simulink model "pmsm_smo"  (R2024b)
settings: Solver=FixedStepDiscrete  StartTime=0.0  StopTime=15  FixedStep=50e-6  RelTol=1e-3  EnableMultiTasking=on
values from neighbouring files (symbols this model uses):
  CalibId = 0    [mchp_pmsm_foc_smo_dsPIC33_data.m]
  CalibIq = 1    [mchp_pmsm_foc_smo_dsPIC33_data.m]
  CalibSpeed = 500    [mchp_pmsm_foc_smo_dsPIC33_data.m]
  CalibTime = 1/CalibFreq    (= 0.12)    [mchp_pmsm_foc_smo_dsPIC33_data.m]
  CalibVd = -0.7    [mchp_pmsm_foc_smo_dsPIC33_data.m]
  CalibVq = 2.69    [mchp_pmsm_foc_smo_dsPIC33_data.m]
  PI_Ki_id = (6.60e2)*Ts    (= 0.033)    [mchp_pmsm_foc_smo_dsPIC33_data.m]
  PI_Ki_iq = (6.60e2)*Ts    (= 0.033)    [mchp_pmsm_foc_smo_dsPIC33_data.m]
  PI_Ki_speed = (1.96e-6)    (= 1.96e-06)    [mchp_pmsm_foc_smo_dsPIC33_data.m]
  PI_Kp_id = 0.852    [mchp_pmsm_foc_smo_dsPIC33_data.m]
  PI_Kp_iq = 0.852    [mchp_pmsm_foc_smo_dsPIC33_data.m]
  PI_Kp_speed = 0.0062756    [mchp_pmsm_foc_smo_dsPIC33_data.m]
  PWM_frequency = 20e3    (= 20000)    [mchp_pmsm_foc_smo_dsPIC33_data.m]
  Ts = T_pwm    (= 5e-05)    [mchp_pmsm_foc_smo_dsPIC33_data.m]
  Ts_serialIn = 100e-3    (= 0.1)    [mchp_pmsm_foc_smo_dsPIC33_data.m]
  Ts_speed = 30*Ts    (= 0.0015)    [mchp_pmsm_foc_smo_dsPIC33_data.m]
undefined symbols (not defined in the file or in its folder): A0, A4, ADC, B0, C10, C11, C6, C7, C8, D11, D12, DiscIntNeverNeededParam, inverter, Max, MaxPer, ms, NumBits1, NumBits2, OpMode, P1, P17, P20, P39, P40, P41, P43, P44, P60, P61, Pin, pmsm, PWM1_Trg1, Resol, s, target, us
libraries: simulink x39, MCHP_Blockset x22, mcbcontrolslib x14, slpidlib x5
(part 4 of 5)

== system pmsm_smo/BOARD MCLV-48V-300W dsPIC33AK128MC106 MC DIM/Downsample Averaged x20 ==
  note: DownSample & Average by changing data scaling
  In1 : Inport
  Compare To Constant : simulink/Logic and Bit Operations/Compare To Constant  relop===  const=1  OutDataTypeStr=boolean
  Counter Limited : simulink/Sources/Counter Limited  uplimit=DownSample-1  tsamp=-1
  Data Type Duplicate : DataTypeDuplicate
  Data Type Propagation : simulink/Signal Attributes/Data Type Propagation  PropDataType=fixdt(1, 16)  IfRefDouble=double  IfRefSingle=single  IsSigned=IsSigned1 or IsSigned2  NumBitsBase=NumBits1+NumBits2  NumBitsMult=1  NumBitsAdd=0  NumBitsAllowFinal=-1  PropScaling=2^-10  ValuesUsedBestPrec=[5 -7]  SlopeBase=Slope1  SlopeMult=1  SlopeAdd=0  BiasBase=Bias1  BiasMult=1  BiasAdd=0
  Data Type Propagation1 : simulink/Signal Attributes/Data Type Propagation  PropDataType=fixdt(1, 16)  IfRefDouble=double  IfRefSingle=single  IsSigned=IsSigned1 or IsSigned2  NumBitsBase=NumBits1+NumBits2  NumBitsMult=1  NumBitsAdd=0  NumBitsAllowFinal=-1  PropScaling=2^-10  ValuesUsedBestPrec=[5 -7]  SlopeBase=PosRange1  SlopeMult=1  SlopeAdd=0  BiasBase=Bias1  BiasMult=1  BiasAdd=0
  Discrete-Time Integrator : DiscreteIntegrator  IntegratorMethod=Accumulation: Backward Euler  gainval=1  ExternalReset=sampled level  SampleTime=-1  OutDataTypeStr=Inherit: Inherit via back propagation  ICPrevOutput=DiscIntNeverNeededParam  ICPrevScaledInput=DiscIntNeverNeededParam
  Gain : Gain  Gain=1/DownSample  OutDataTypeStr=Inherit: Inherit via back propagation  RndMeth=Round
  Gain1 : Gain  Gain=1/DownSample  OutDataTypeStr=Inherit: Inherit via back propagation
  Rate Transition1 : RateTransition  OutPortSampleTimeOpt=Multiple of input port sample time  OutPortSampleTimeMultiple=DownSample  OutPortSampleTime=DownSample
  Rate Transition3 : RateTransition  OutPortSampleTimeOpt=Multiple of input port sample time  OutPortSampleTimeMultiple=DownSample  OutPortSampleTime=DownSample
  Terminator : Terminator
  Out1 : Outport  VectorParamsAs1DForOutWhenUnconnected=off
  wires:
  Gain1/1 -> Data Type Propagation1/3, Terminator/1
  Rate Transition1/1 -> Data Type Duplicate/1, Data Type Propagation1/1, Data Type Propagation1/2
  Gain/1 -> Out1/1, Data Type Duplicate/2
  Counter Limited/1 -> Compare To Constant/1
  Discrete-Time Integrator/1 -> Rate Transition3/1, Data Type Propagation/3
  Compare To Constant/1 -> Discrete-Time Integrator/2
  In1/1 -> Data Type Propagation/1, Data Type Propagation/2, Discrete-Time Integrator/1, Rate Transition1/1
  Rate Transition3/1 -> Gain/1, Gain1/1

== system pmsm_smo/BOARD MCLV-48V-300W dsPIC33AK128MC106 MC DIM/Downsample x20 ==
  note: DownSample & Average by changing data scaling
  In1 : Inport
  Compare To Constant : simulink/Logic and Bit Operations/Compare To Constant  relop===  const=1  OutDataTypeStr=boolean
  Counter Limited : simulink/Sources/Counter Limited  uplimit=DownSample-1  tsamp=-1
  Data Type Duplicate : DataTypeDuplicate
  Data Type Propagation : simulink/Signal Attributes/Data Type Propagation  PropDataType=fixdt(1, 16)  IfRefDouble=double  IfRefSingle=single  IsSigned=IsSigned1 or IsSigned2  NumBitsBase=NumBits1+NumBits2  NumBitsMult=1  NumBitsAdd=0  NumBitsAllowFinal=-1  PropScaling=2^-10  ValuesUsedBestPrec=[5 -7]  SlopeBase=Slope1  SlopeMult=1  SlopeAdd=0  BiasBase=Bias1  BiasMult=1  BiasAdd=0
  Data Type Propagation1 : simulink/Signal Attributes/Data Type Propagation  PropDataType=fixdt(1, 16)  IfRefDouble=double  IfRefSingle=single  IsSigned=IsSigned1 or IsSigned2  NumBitsBase=NumBits1+NumBits2  NumBitsMult=1  NumBitsAdd=0  NumBitsAllowFinal=-1  PropScaling=2^-10  ValuesUsedBestPrec=[5 -7]  SlopeBase=PosRange1  SlopeMult=1  SlopeAdd=0  BiasBase=Bias1  BiasMult=1  BiasAdd=0
  Discrete-Time Integrator : DiscreteIntegrator  IntegratorMethod=Accumulation: Backward Euler  gainval=1  ExternalReset=sampled level  SampleTime=-1  OutDataTypeStr=Inherit: Inherit via back propagation  ICPrevOutput=DiscIntNeverNeededParam  ICPrevScaledInput=DiscIntNeverNeededParam
  Gain : Gain  Gain=1/DownSample  OutDataTypeStr=Inherit: Inherit via back propagation  RndMeth=Round
  Gain1 : Gain  Gain=1/DownSample  OutDataTypeStr=Inherit: Inherit via back propagation
  Rate Transition1 : RateTransition  OutPortSampleTimeOpt=Multiple of input port sample time  OutPortSampleTimeMultiple=DownSample  OutPortSampleTime=DownSample
  Rate Transition3 : RateTransition  OutPortSampleTimeOpt=Multiple of input port sample time  OutPortSampleTimeMultiple=DownSample  OutPortSampleTime=DownSample
  Terminator : Terminator
  Out1 : Outport  VectorParamsAs1DForOutWhenUnconnected=off
  wires:
  Rate Transition3/1 -> Gain1/1, Gain/1
  In1/1 -> Rate Transition1/1, Discrete-Time Integrator/1, Data Type Propagation/2, Data Type Propagation/1
  Compare To Constant/1 -> Discrete-Time Integrator/2
  Discrete-Time Integrator/1 -> Data Type Propagation/3, Rate Transition3/1
  Counter Limited/1 -> Compare To Constant/1
  Gain/1 -> Data Type Duplicate/2, Out1/1
  Rate Transition1/1 -> Data Type Propagation1/2, Data Type Propagation1/1, Data Type Duplicate/1
  Gain1/1 -> Terminator/1, Data Type Propagation1/3

== system pmsm_smo/BOARD MCLV-48V-300W dsPIC33AK128MC106 MC DIM/Downsample x20 _ ==
  note: DownSample & Average by changing data scaling
  In1 : Inport
  Compare To Constant : simulink/Logic and Bit Operations/Compare To Constant  relop===  const=1  OutDataTypeStr=boolean
  Counter Limited : simulink/Sources/Counter Limited  uplimit=DownSample-1  tsamp=-1
  Data Type Duplicate : DataTypeDuplicate
  Data Type Propagation : simulink/Signal Attributes/Data Type Propagation  PropDataType=fixdt(1, 16)  IfRefDouble=double  IfRefSingle=single  IsSigned=IsSigned1 or IsSigned2  NumBitsBase=NumBits1+NumBits2  NumBitsMult=1  NumBitsAdd=0  NumBitsAllowFinal=-1  PropScaling=2^-10  ValuesUsedBestPrec=[5 -7]  SlopeBase=Slope1  SlopeMult=1  SlopeAdd=0  BiasBase=Bias1  BiasMult=1  BiasAdd=0
  Data Type Propagation1 : simulink/Signal Attributes/Data Type Propagation  PropDataType=fixdt(1, 16)  IfRefDouble=double  IfRefSingle=single  IsSigned=IsSigned1 or IsSigned2  NumBitsBase=NumBits1+NumBits2  NumBitsMult=1  NumBitsAdd=0  NumBitsAllowFinal=-1  PropScaling=2^-10  ValuesUsedBestPrec=[5 -7]  SlopeBase=PosRange1  SlopeMult=1  SlopeAdd=0  BiasBase=Bias1  BiasMult=1  BiasAdd=0
  Discrete-Time Integrator : DiscreteIntegrator  IntegratorMethod=Accumulation: Backward Euler  gainval=1  ExternalReset=sampled level  SampleTime=-1  OutDataTypeStr=Inherit: Inherit via back propagation  ICPrevOutput=DiscIntNeverNeededParam  ICPrevScaledInput=DiscIntNeverNeededParam
  Gain : Gain  Gain=1/DownSample  OutDataTypeStr=Inherit: Inherit via back propagation  RndMeth=Round
  Gain1 : Gain  Gain=1/DownSample  OutDataTypeStr=Inherit: Inherit via back propagation
  Rate Transition1 : RateTransition  OutPortSampleTimeOpt=Multiple of input port sample time  OutPortSampleTimeMultiple=DownSample  OutPortSampleTime=DownSample
  Rate Transition3 : RateTransition  OutPortSampleTimeOpt=Multiple of input port sample time  OutPortSampleTimeMultiple=DownSample  OutPortSampleTime=DownSample
  Terminator : Terminator
  Out1 : Outport  VectorParamsAs1DForOutWhenUnconnected=off
  wires:
  Gain1/1 -> Data Type Propagation1/3, Terminator/1
  Rate Transition1/1 -> Data Type Duplicate/1, Data Type Propagation1/1, Data Type Propagation1/2
  Gain/1 -> Out1/1, Data Type Duplicate/2
  Counter Limited/1 -> Compare To Constant/1
  Discrete-Time Integrator/1 -> Rate Transition3/1, Data Type Propagation/3
  Compare To Constant/1 -> Discrete-Time Integrator/2
  In1/1 -> Data Type Propagation/1, Data Type Propagation/2, Discrete-Time Integrator/1, Rate Transition1/1
  Rate Transition3/1 -> Gain/1, Gain1/1

== system pmsm_smo/BOARD MCLV-48V-300W dsPIC33AK128MC106 MC DIM/MCLV 48V-300W board webpage ==

== system pmsm_smo/BOARD MCLV-48V-300W dsPIC33AK128MC106 MC DIM/Timing Analysis ==
  note: CPU overload is 0 if no overload took place between two MCU Overload block execution.
      | Otherwise, bits field output code for TID(s) responsible for at least one overload.
  Downsample Averaged2 : Subsystem  mask{InputSampleTime=.0005, DownSample=200}
      mask prompts: InputSampleTime "Input sample time"; DownSample "DownSample Factor"
  Gain : Gain  Gain=5e-9/.0005 * 100  OutMin=0  OutMax=100  OutDataTypeStr=fixdt(0,16)  RndMeth=Simplest  SaturateOnIntegerOverflow=on
  MCU Load : MCHP_Blockset/Profiling/MCU Load  MCULoadPin_TXT=None  MCULoadMeasure=on  TIMER_Resolution_TXT="Resol: 0.005(us)  -  Max: 0.328(ms)"  MCHP_TIMER_REQUEST={MCU_Load}{MCU_Load}21:5:0:0:[]:32768;  MCHP_TIMER_RESULT=[2 65535 ]  MCHP_MASTERLINK=pmsm_smo/BOARD MCLV-48V-300W dsPIC33AK128MC106 MC DIM/Microchip Master  MCHP_COMPILED_INFO="CompiledSampleTime= [0.00050000000000000001041   0 ];CompiledInportDataTypes=[    ];CompiledInportDataWidth=[];"  Info="Timer 2:  Resol: 5(ns)  -  Max: 327.68(us)"  SampleTime=.0005
      settings: SourceProductName=MPLAB Device Blocks for Simulink
  MCU Overload : MCHP_Blockset/Profiling/MCU Overload  MCUOverloadBlockOutput=on  MCUOverLoadPin_TXT=None  MCHP_MASTERLINK=pmsm_smo/BOARD MCLV-48V-300W dsPIC33AK128MC106 MC DIM/Microchip Master  SampleTime=-1
      settings: SourceProductName=MPLAB Device Blocks for Simulink
  Overload : Constant  Value=65535  OutDataTypeStr=Inherit: Inherit via back propagation
  Rate Transition : RateTransition  Deterministic=off  OutPortSampleTime=.0005*200
  Switch : Switch  Criteria=u2 ~= 0  SaturateOnIntegerOverflow=off  InputSameDT=off
  CPU Load : Outport  Unit=%  SampleTime=.0005*200
  CPU Overload : Outport  Port=2
  wires:
  Rate Transition/1 -> Switch/2
  MCU Overload/1 -> Rate Transition/1, CPU Overload/1
  MCU Load/1 -> Downsample Averaged2/1(In1)
  Downsample Averaged2/1(Out1) -> Switch/3
  Switch/1 -> Gain/1
  Overload/1 -> Switch/1
  Gain/1 -> CPU Load/1

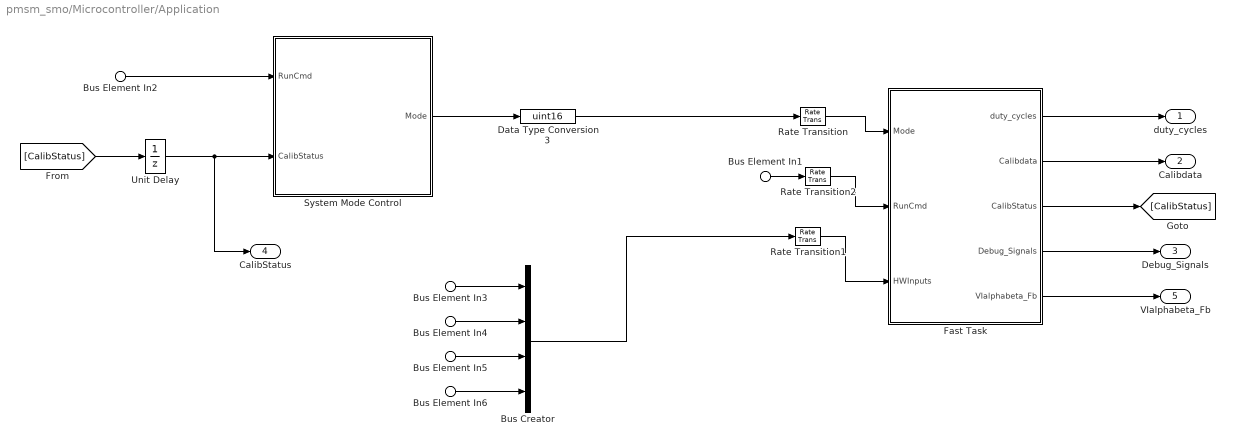
== system pmsm_smo/Microcontroller/Application ==
  Bus Element In3 : Inport  PortName=Currents  Element=Iab
  Bus Element In4 : Inport  Port=2  PortName=PositionAndSpeed  Element=Theta_SMO
  Bus Element In6 : Inport  Port=2  PortName=PositionAndSpeed  Element=Speed_SMO
  Bus Element In1 : Inport  Port=3  PortName=Commands  Element=RunCmd
  Bus Element In2 : Inport  Port=3  PortName=Commands  Element=RunCmd
  Bus Element In5 : Inport  Port=3  PortName=Commands  Element=SpeedRef
  Bus Creator : BusCreator  Inputs=4
  Data Type Conversion3 : DataTypeConversion  OutDataTypeStr=uint16  RndMeth=Simplest  SaturateOnIntegerOverflow=off
  Fast Task : Subsystem
  Rate Transition : RateTransition  Deterministic=off  OutPortSampleTime=Ts
  Rate Transition1 : RateTransition  Deterministic=off  OutPortSampleTime=Ts
  Rate Transition2 : RateTransition  Deterministic=off  OutPortSampleTime=Ts
  System Mode Control : Subsystem
  Unit Delay : UnitDelay  SampleTime=-1  HasFrameUpgradeWarning=on
  duty_cycles : Outport  VectorParamsAs1DForOutWhenUnconnected=off
  Calibdata : Outport  Port=2
  Debug_Signals : Outport  Port=3
  CalibStatus : Outport  Port=4
  VIalphabeta_Fb : Outport  Port=5
  wires:
  System Mode Control/1(Mode) -> Data Type Conversion3/1
  Data Type Conversion3/1 -> Rate Transition/1
  Rate Transition/1 -> Fast Task/1(Mode)
  Bus Element In1/1 -> Rate Transition2/1
  Fast Task/1(duty_cycles) -> duty_cycles/1
  Bus Element In2/1 -> System Mode Control/1(RunCmd)
  Fast Task/3(CalibStatus) -> [CalibStatus]
  [CalibStatus] -> Unit Delay/1
  Bus Element In3/1 -> Bus Creator/1
  Bus Element In4/1 -> Bus Creator/2
  Bus Element In5/1 -> Bus Creator/3
  Bus Element In6/1 -> Bus Creator/4
  Bus Creator/1 -> Rate Transition1/1
  Rate Transition1/1 -> Fast Task/3(HWInputs)
  Rate Transition2/1 -> Fast Task/2(RunCmd)
  Unit Delay/1 -> CalibStatus/1, System Mode Control/2(CalibStatus)
  Fast Task/2(Calibdata) -> Calibdata/1
  Fast Task/4(Debug_Signals) -> Debug_Signals/1
  Fast Task/5(VIalphabeta_Fb) -> VIalphabeta_Fb/1

== system pmsm_smo/Microcontroller/Application_Abstraction ==
  Iab_Measured : Inport
  calibdata : Inport  Port=2
  VIalphabeta_Fb : Inport  Port=3
  Commands : Inport  Port=4
  Bus Creator : BusCreator  Inputs=1
  Bus Creator1 : BusCreator  Inputs=2
  SMO : Subsystem
  Currents : Outport
  PositionAndSpeed : Outport  Port=2
  wires:
  Bus Creator1/1 -> PositionAndSpeed/1
  Iab_Measured/1 -> Bus Creator/1  "Iab"
  Bus Creator/1 -> Currents/1
  Commands/1 -> SMO/2(Commands)
  VIalphabeta_Fb/1 -> SMO/1(VIalphabeta_Fb)
  SMO/1(Speed_meas) -> Bus Creator1/1  "Speed_SMO"
  SMO/2(Pos_PU) -> Bus Creator1/2  "Theta_SMO"
  calibdata/1 -> SMO/3(calibdata)

== system pmsm_smo/Microcontroller/Command_Signals ==
  note: Subsystem
  Command_Data : Inport
  Bus Creator : BusCreator  Inputs=2
  Command Signals : Subsystem  Variant=on  VariantControlMode=sim codegen switching
  Commands : Outport
  wires:
  Bus Creator/1 -> Commands/1
  Command Signals/1(RunCmd) -> Bus Creator/1  "RunCmd"
  Command Signals/2(SpeedRef) -> Bus Creator/2  "SpeedRef"
  Command_Data/1 -> Command Signals/1(Command_Data)

== system pmsm_smo/Microcontroller/Data Monitoring ==
  Data_Monitor : Inport
  Constant : Constant  OutDataTypeStr=boolean
  Rate Transition13 : RateTransition  Deterministic=off  OutPortSampleTime=Ts_serialIn
  Rate Transition14 : RateTransition  Deterministic=off  OutPortSampleTime=Ts_serialOut
  Rate Transition15 : RateTransition  Deterministic=off  OutPortSampleTime=Ts_serialOut
  SerialInDrivers : Subsystem
  SerialOutDrivers : Subsystem  Variant=on  VariantControlMode=sim codegen switching
  Subsystem Reference : Subsystem  TreatAsAtomicUnit=on  ReferencedSubsystem=SCIOutAbstractionFocQep
  Subsystem Reference1 : Subsystem  TreatAsAtomicUnit=on  ReferencedSubsystem=SCIInAbstractionFocQep
  Terminator : Terminator
  wires:
  Subsystem Reference1/1 -> Terminator/1
  Constant/1 -> Rate Transition13/1
  Rate Transition15/1 -> Subsystem Reference/1
  Rate Transition14/1 -> Subsystem Reference/2
  Subsystem Reference1/2 -> Rate Transition15/1
  Rate Transition13/1 -> Subsystem Reference1/2
  Subsystem Reference/1 -> SerialOutDrivers/1(SerialData)
  SerialInDrivers/1(SCI_Data) -> Subsystem Reference1/1  "sci data 8 bytes"
  Data_Monitor/1 -> Rate Transition14/1

== system pmsm_smo/Microcontroller/Sensor_Signals ==
  note: 1) Add Subsystem or Model blocks as valid variant choices.
      | 2) You cannot connect blocks at this level. At simulation, connectivity is automatically
      | determined, based on the active variant and port name matching.
  Sim_In : Inport
  Codegen_in : Inport  Port=2
  Codegen : Subsystem  VariantControl=(codegen)
  sim : Subsystem  VariantControl=(sim)
  Sensor_signals : Outport

== system pmsm_smo/BOARD MCLV-48V-300W dsPIC33AK128MC106 MC DIM/Center & sign reversal/Downsample Averaged 2000 samples remove bias ==
  note: DownSample & Average by changing data scaling
  In1 : Inport
  Enable : EnablePort
  Compare To Constant : simulink/Logic and Bit Operations/Compare To Constant  relop===  const=1  OutDataTypeStr=boolean
  Counter Limited : simulink/Sources/Counter Limited  uplimit=DownSample-1  tsamp=-1
  Data Type Duplicate : DataTypeDuplicate
  Data Type Propagation : simulink/Signal Attributes/Data Type Propagation  PropDataType=fixdt(1, 16)  IfRefDouble=double  IfRefSingle=single  IsSigned=IsSigned1 or IsSigned2  NumBitsBase=NumBits1+NumBits2  NumBitsMult=1  NumBitsAdd=0  NumBitsAllowFinal=-1  PropScaling=2^-10  ValuesUsedBestPrec=[5 -7]  SlopeBase=Slope1  SlopeMult=1  SlopeAdd=0  BiasBase=Bias1  BiasMult=1  BiasAdd=0
  Data Type Propagation1 : simulink/Signal Attributes/Data Type Propagation  PropDataType=fixdt(1, 16)  IfRefDouble=double  IfRefSingle=single  IsSigned=IsSigned1 or IsSigned2  NumBitsBase=NumBits1+NumBits2  NumBitsMult=1  NumBitsAdd=0  NumBitsAllowFinal=-1  PropScaling=2^-10  ValuesUsedBestPrec=[5 -7]  SlopeBase=PosRange1  SlopeMult=1  SlopeAdd=0  BiasBase=Bias1  BiasMult=1  BiasAdd=0
  Discrete-Time Integrator : DiscreteIntegrator  IntegratorMethod=Accumulation: Backward Euler  gainval=1  ExternalReset=sampled level  SampleTime=-1  OutDataTypeStr=Inherit: Inherit via back propagation  ICPrevOutput=DiscIntNeverNeededParam  ICPrevScaledInput=DiscIntNeverNeededParam
  Gain : Gain  Gain=1/DownSample  OutDataTypeStr=uint16  RndMeth=Round
  Gain1 : Gain  Gain=1/DownSample  OutDataTypeStr=Inherit: Inherit via back propagation
  Gain2 : Gain  OutDataTypeStr=int32
  Rate Transition1 : RateTransition  OutPortSampleTimeOpt=Multiple of input port sample time  OutPortSampleTimeMultiple=DownSample  OutPortSampleTime=DownSample
  Rate Transition3 : RateTransition  OutPortSampleTimeOpt=Multiple of input port sample time  OutPortSampleTimeMultiple=DownSample  OutPortSampleTime=DownSample
  Terminator : Terminator
  Out1 : Outport  InitialOutput=[32768]  VectorParamsAs1DForOutWhenUnconnected=off
  wires:
  Gain1/1 -> Gain2/1, Data Type Propagation1/3  "Offset"
  Rate Transition1/1 -> Data Type Duplicate/1, Data Type Propagation1/1, Data Type Propagation1/2
  Gain/1 -> Terminator/1, Data Type Duplicate/2  "Offset_Value_Uint16"
  Counter Limited/1 -> Compare To Constant/1
  Discrete-Time Integrator/1 -> Rate Transition3/1, Data Type Propagation/3  "Intergrator_Out"
  Compare To Constant/1 -> Discrete-Time Integrator/2
  In1/1 -> Data Type Propagation/1, Data Type Propagation/2, Discrete-Time Integrator/1, Rate Transition1/1
  Rate Transition3/1 -> Gain/1, Gain1/1
  Gain2/1 -> Out1/1  "Offset_Value_int32"

== system pmsm_smo/BOARD MCLV-48V-300W dsPIC33AK128MC106 MC DIM/Timing Analysis/Downsample Averaged2 ==
  note: DownSample & Average by changing data scaling
  In1 : Inport
  Compare To Constant : simulink/Logic and Bit Operations/Compare To Constant  relop===  const=1  OutDataTypeStr=boolean
  Counter Limited : simulink/Sources/Counter Limited  uplimit=DownSample-1  tsamp=-1
  Data Type Duplicate : DataTypeDuplicate
  Data Type Propagation : simulink/Signal Attributes/Data Type Propagation  PropDataType=fixdt(1, 16)  IfRefDouble=double  IfRefSingle=single  IsSigned=IsSigned1 or IsSigned2  NumBitsBase=NumBits1+NumBits2  NumBitsMult=1  NumBitsAdd=0  NumBitsAllowFinal=-1  PropScaling=2^-10  ValuesUsedBestPrec=[5 -7]  SlopeBase=Slope1  SlopeMult=1  SlopeAdd=0  BiasBase=Bias1  BiasMult=1  BiasAdd=0
  Data Type Propagation1 : simulink/Signal Attributes/Data Type Propagation  PropDataType=fixdt(1, 16)  IfRefDouble=double  IfRefSingle=single  IsSigned=IsSigned1 or IsSigned2  NumBitsBase=NumBits1+NumBits2  NumBitsMult=1  NumBitsAdd=0  NumBitsAllowFinal=-1  PropScaling=2^-10  ValuesUsedBestPrec=[5 -7]  SlopeBase=PosRange1  SlopeMult=1  SlopeAdd=0  BiasBase=Bias1  BiasMult=1  BiasAdd=0
  Discrete-Time Integrator : DiscreteIntegrator  IntegratorMethod=Accumulation: Backward Euler  gainval=1  ExternalReset=sampled level  SampleTime=-1  OutDataTypeStr=Inherit: Inherit via back propagation  ICPrevOutput=DiscIntNeverNeededParam  ICPrevScaledInput=DiscIntNeverNeededParam
  Gain : Gain  Gain=1/DownSample  OutDataTypeStr=Inherit: Inherit via back propagation
  Gain1 : Gain  Gain=1/DownSample  OutDataTypeStr=Inherit: Inherit via back propagation
  Rate Transition1 : RateTransition  Deterministic=off  OutPortSampleTime=[InputSampleTime * DownSample]
  Rate Transition3 : RateTransition  OutPortSampleTime=[InputSampleTime * DownSample]
  Terminator : Terminator
  Out1 : Outport  VectorParamsAs1DForOutWhenUnconnected=off
  wires:
  Rate Transition3/1 -> Gain1/1, Gain/1
  In1/1 -> Discrete-Time Integrator/1, Rate Transition1/1, Data Type Propagation/2, Data Type Propagation/1
  Compare To Constant/1 -> Discrete-Time Integrator/2
  Discrete-Time Integrator/1 -> Data Type Propagation/3, Rate Transition3/1
  Counter Limited/1 -> Compare To Constant/1
  Gain/1 -> Data Type Duplicate/2, Out1/1
  Rate Transition1/1 -> Data Type Propagation1/2, Data Type Propagation1/1, Data Type Duplicate/1
  Gain1/1 -> Data Type Propagation1/3, Terminator/1

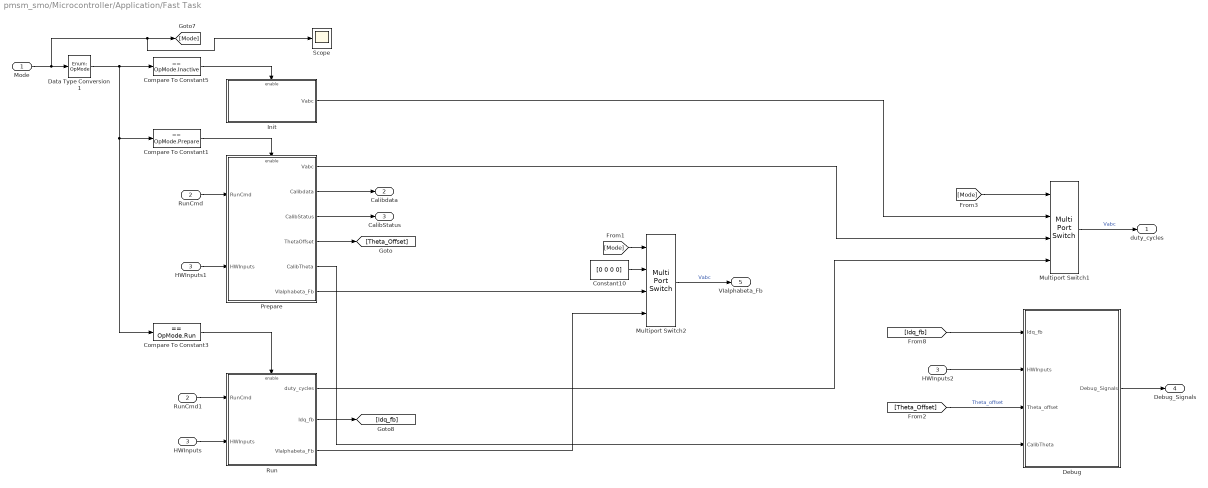
== system pmsm_smo/Microcontroller/Application/Fast Task ==
  Mode : Inport
  RunCmd : Inport  Port=2
  HWInputs : Inport  Port=3
  Compare To Constant1 : simulink/Logic and Bit Operations/Compare To Constant  relop===  const=OpMode.Prepare  OutDataTypeStr=boolean
  Compare To Constant3 : simulink/Logic and Bit Operations/Compare To Constant  relop===  const=OpMode.Run  OutDataTypeStr=boolean
  Compare To Constant5 : simulink/Logic and Bit Operations/Compare To Constant  relop===  const=OpMode.Inactive  OutDataTypeStr=boolean
  Constant10 : Constant  Value=[0 0 0 0]  OutDataTypeStr=dataType  SampleTime=Ts
  Data Type Conversion1 : DataTypeConversion  OutDataTypeStr=Enum: OpMode  RndMeth=Simplest  SaturateOnIntegerOverflow=off
  Debug : Subsystem
  HWInputs1 : InportShadow  Port=3
  HWInputs2 : InportShadow  Port=3
  Init : Subsystem
  Multiport Switch1 : MultiPortSwitch  DataPortOrder=Zero-based contiguous  DiagnosticForDefault=None  zeroidx=on  OutDataTypeStr=single  SaturateOnIntegerOverflow=off  InputSameDT=off
  Multiport Switch2 : MultiPortSwitch  DataPortOrder=Zero-based contiguous  DiagnosticForDefault=None  zeroidx=on  OutDataTypeStr=single  SaturateOnIntegerOverflow=off  InputSameDT=off
  Prepare : Subsystem
  Run : Subsystem
  RunCmd1 : InportShadow  Port=2
  Scope : Scope
  duty_cycles : Outport
  Calibdata : Outport  Port=2
  CalibStatus : Outport  Port=3
  Debug_Signals : Outport  Port=4
  VIalphabeta_Fb : Outport  Port=5
  wires:
  RunCmd/1 -> Prepare/1(RunCmd)
  Compare To Constant5/1 -> Init/Enable
  Mode/1 -> Scope/1, [Mode], Data Type Conversion1/1
  Compare To Constant1/1 -> Prepare/Enable
  [Mode] -> Multiport Switch1/1
  Init/1(Vabc) -> Multiport Switch1/2
  HWInputs/1 -> Run/2(HWInputs)
  RunCmd1/1 -> Run/1(RunCmd)
  Multiport Switch1/1 -> duty_cycles/1  "Vabc"
  Data Type Conversion1/1 -> Compare To Constant5/1, Compare To Constant3/1, Compare To Constant1/1
  Compare To Constant3/1 -> Run/Enable
  HWInputs2/1 -> Debug/2(HWInputs)
  Debug/1(Debug_Signals) -> Debug_Signals/1
  Run/1(duty_cycles) -> Multiport Switch1/4
  Prepare/1(Vabc) -> Multiport Switch1/3
  HWInputs1/1 -> Prepare/2(HWInputs)
  Run/2(Idq_fb) -> [Idq_fb]
  [Idq_fb] -> Debug/1(Idq_fb)
  Prepare/2(Calibdata) -> Calibdata/1
  Prepare/4(ThetaOffset) -> [Theta_Offset]
  Prepare/3(CalibStatus) -> CalibStatus/1
  [Theta_Offset] -> Debug/3(Theta_offset)  "Theta_offset"
  Prepare/5(CalibTheta) -> Debug/4(CalibTheta)
  [Mode] -> Multiport Switch2/1
  Multiport Switch2/1 -> VIalphabeta_Fb/1  "Vabc"
  Constant10/1 -> Multiport Switch2/2
  Prepare/6(VIalphabeta_Fb) -> Multiport Switch2/3
  Run/3(VIalphabeta_Fb) -> Multiport Switch2/4

== system pmsm_smo/Microcontroller/Application/System Mode Control ==
  RunCmd : Inport
  CalibStatus : Inport  Port=2
  Data Store Write : DataStoreWrite  DataStoreName=CurrOffsetMeas  IndexOptions=Index vector (dialog)  Indices=1  OutputSizes=1
  System Control : Stateflow chart  TreatAsAtomicUnit=on
  Mode : Outport
  wires:
  RunCmd/1 -> System Control/1(RunCmd)
  CalibStatus/1 -> System Control/2(MotorReady)
  System Control/1(Mode) -> Mode/1
  System Control/2(CurrOffsetMeas) -> Data Store Write/1

== system pmsm_smo/Microcontroller/Application_Abstraction/SMO ==
  VIalphabeta_Fb : Inport
  Bus Element In : Inport  Port=2  PortName=Commands  Element=SpeedRef
  calibdata : Inport  Port=3
  Demux : Demux
  Rate Transition2 : RateTransition  Deterministic=off
  Sliding Mode Observer : Subsystem
  Speed_meas : Outport
  Pos_PU : Outport  Port=2
  wires:
  VIalphabeta_Fb/1 -> Demux/1
  Demux/4 -> Sliding Mode Observer/4(Vbeta_PU)
  Demux/2 -> Sliding Mode Observer/2(Ibeta_PU)
  Demux/1 -> Sliding Mode Observer/1(Ialpha_PU)
  Demux/3 -> Sliding Mode Observer/3(Valpha_PU)
  Sliding Mode Observer/2(west) -> Speed_meas/1
  Bus Element In/1 -> Rate Transition2/1
  Rate Transition2/1 -> Sliding Mode Observer/5(SpeedRef_PU)
  Sliding Mode Observer/1(theta) -> Pos_PU/1
  calibdata/1 -> Sliding Mode Observer/6(calibdata)

== system pmsm_smo/Microcontroller/Command_Signals/Command Signals ==
  Command_Data : Inport
  Codegen : Subsystem  VariantControl=(codegen)
  Sim : Subsystem  VariantControl=(sim)
  RunCmd : Outport
  SpeedRef : Outport  Port=2

== system pmsm_smo/Microcontroller/Data Monitoring/SerialInDrivers ==
  Compare To Constant : simulink/Logic and Bit Operations/Compare To Constant  relop=>=  const=8  OutDataTypeStr=boolean
  Data Type Conversion : DataTypeConversion  SaturateOnIntegerOverflow=off  RndMeth=Floor
  Triggered Subsystem : Subsystem  TreatAsAtomicUnit=on
  UART Rx : MCHP_Blockset/BUS UART/UART Rx  UART_REF=1  Flag_Out=on  Rx_Size_popup=User defined  Rx_Size=8  S_Rx_Size=8  Split=Read all received char  SplitChar=10  OutputDefault_popup=do nothing (end of output vector will be undefined)  OutputDefault=-1  ORDERING=None  SampleTime=Ts_serialIn  MCHP_MASTERLINK=pmsm_smo/BOARD MCLV-48V-300W dsPIC33AK128MC106 MC DIM/Microchip Master  MCHP_COMPILED_INFO="CompiledSampleTime= [0.10000000000000000555   0 ];CompiledInportDataTypes=[    ];CompiledInportDataWidth=[];"
      settings: SourceProductName=MPLAB Device Blocks for Simulink
  SCI_Data : Outport
  wires:
  Compare To Constant/1 -> Triggered Subsystem/Trigger
  UART Rx/1 -> Data Type Conversion/1
  UART Rx/2 -> Triggered Subsystem/1(In1)
  Triggered Subsystem/1(SCI_Data) -> SCI_Data/1
  Data Type Conversion/1 -> Compare To Constant/1

== system pmsm_smo/Microcontroller/Data Monitoring/SerialOutDrivers ==
  SerialData : Inport
  codegen : Subsystem  VariantControl=(codegen)
  sim : Subsystem  VariantControl=(sim)

== system pmsm_smo/Microcontroller/Sensor_Signals/Codegen ==
  Sim_In : Inport
  Codegen_in : Inport  Port=2
  Terminator : Terminator
  Sensor_signals : Outport
  wires:
  Sim_In/1 -> Terminator/1
  Codegen_in/1 -> Sensor_signals/1

== system pmsm_smo/Microcontroller/Sensor_Signals/sim ==
  Sim_In : Inport
  Codegen_in : Inport  Port=2
  Terminator : Terminator
  Sensor_signals : Outport
  wires:
  Sim_In/1 -> Sensor_signals/1
  Codegen_in/1 -> Terminator/1

== system pmsm_smo/Microcontroller/Application/Fast Task/Debug ==
  Idq_fb : Inport
  HWInputs : Inport  Port=2
  Theta_offset : Inport  Port=3
  CalibTheta : Inport  Port=4
  Bus Creator : BusCreator  Inputs=7
  Bus Selector : BusSelector  OutputSignals=SpeedRef,Speed_SMO,Iab,Theta_SMO
  Demux : Demux
  Mux : Mux
  Debug_Signals : Outport
  wires:
  Idq_fb/1 -> Demux/1
  Bus Selector/2 -> Bus Creator/2  "<Speed_SMO>"
  Bus Selector/1 -> Bus Creator/1  "<SpeedRef>"
  Demux/2 -> Mux/2  "Id_fb"
  HWInputs/1 -> Bus Selector/1
  Demux/1 -> Mux/1  "Id_ref"
  Demux/3 -> Mux/3  "Iq_ref"
  Demux/4 -> Mux/4  "Iq_fb"
  Bus Selector/3 -> Bus Creator/3  "<Iab>"
  Bus Creator/1 -> Debug_Signals/1
  Bus Selector/4 -> Bus Creator/4  "<Theta_SMO>"
  Mux/1 -> Bus Creator/5  "Idq"
  Theta_offset/1 -> Bus Creator/6  "Theta_offset"
  CalibTheta/1 -> Bus Creator/7

== system pmsm_smo/Microcontroller/Application/Fast Task/Init ==
  Enable : EnablePort
  Constant10 : Constant  Value=[0 0 0]  OutDataTypeStr=dataType  SampleTime=Ts
  Vabc : Outport
  wires:
  Constant10/1 -> Vabc/1

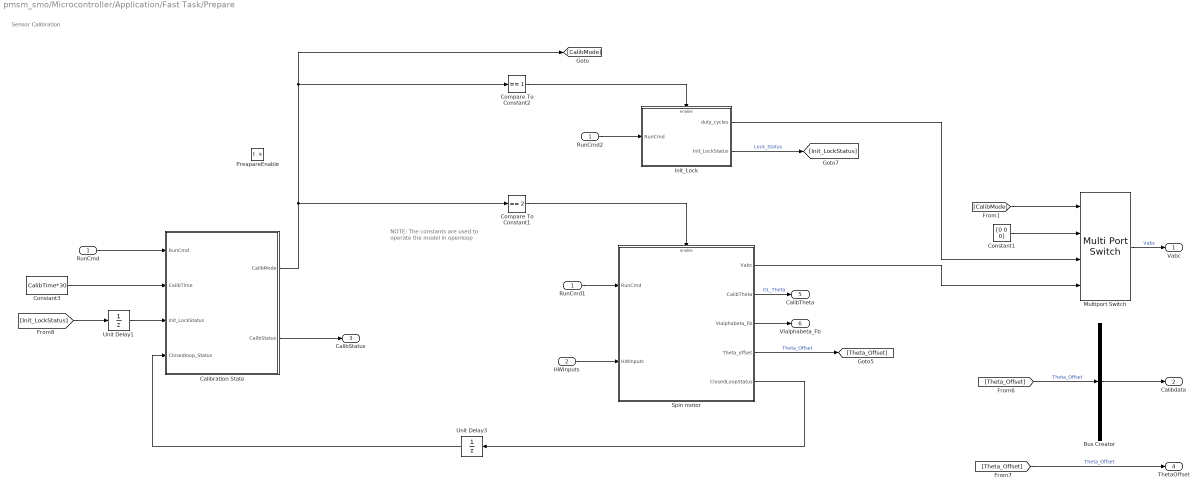
== system pmsm_smo/Microcontroller/Application/Fast Task/Prepare ==
  note: Sensor Calibration
  note: NOTE:
      | The constants are used to operate
      | the model in openloop
  RunCmd : Inport
  HWInputs : Inport  Port=2
  PreapareEnable : EnablePort
  Bus Creator : BusCreator  Inputs=1
  Calibration State : Stateflow chart  TreatAsAtomicUnit=on
  Compare To Constant1 : simulink/Logic and Bit Operations/Compare To Constant  relop===  const=2  OutDataTypeStr=boolean
  Compare To Constant2 : simulink/Logic and Bit Operations/Compare To Constant  relop===  const=1  OutDataTypeStr=boolean
  Constant1 : Constant  Value=[0 0 0]  OutDataTypeStr=dataType  SampleTime=Ts
  Constant3 : Constant  Value=CalibTime*30  OutDataTypeStr=single  SampleTime=Ts
  Init_Lock : Subsystem
  Multiport Switch : MultiPortSwitch  DataPortOrder=Zero-based contiguous  zeroidx=on  SaturateOnIntegerOverflow=off  InputSameDT=off
  RunCmd1 : InportShadow
  RunCmd2 : InportShadow
  Spin motor : Subsystem
  Unit Delay1 : UnitDelay  SampleTime=-1  HasFrameUpgradeWarning=on
  Unit Delay3 : UnitDelay  SampleTime=-1  HasFrameUpgradeWarning=on
  Vabc : Outport  VectorParamsAs1DForOutWhenUnconnected=off
  Calibdata : Outport  Port=2
  CalibStatus : Outport  Port=3
  ThetaOffset : Outport  Port=4
  CalibTheta : Outport  Port=5
  VIalphabeta_Fb : Outport  Port=6
  wires:
  Bus Creator/1 -> Calibdata/1
  Constant1/1 -> Multiport Switch/2
  Compare To Constant1/1 -> Spin motor/Enable
  [CalibMode] -> Multiport Switch/1
  Calibration State/1(CalibMode) -> Compare To Constant2/1, [CalibMode], Compare To Constant1/1
  Calibration State/2(CalibStatus) -> CalibStatus/1
  Multiport Switch/1 -> Vabc/1  "Vabc"
  [Theta_Offset] -> Bus Creator/1  "Theta_Offset"
  [Theta_Offset] -> ThetaOffset/1  "Theta_Offset"
  Spin motor/2(CalibTheta) -> CalibTheta/1  "OL_Theta"
  Compare To Constant2/1 -> Init_Lock/Enable
  Init_Lock/2(Init_LockStatus) -> [Init_LockStatus]  "Lock_Status"
  [Init_LockStatus] -> Unit Delay1/1
  Init_Lock/1(duty_cycles) -> Multiport Switch/3
  Spin motor/1(Vabc) -> Multiport Switch/4
  Spin motor/5(ClosedLoopStatus) -> Unit Delay3/1
  RunCmd1/1 -> Spin motor/1(RunCmd)
  HWInputs/1 -> Spin motor/2(HWInputs)
  Spin motor/3(VIalphabeta_Fb) -> VIalphabeta_Fb/1
  Spin motor/4(Theta_offset) -> [Theta_Offset]  "Theta_Offset"
  RunCmd2/1 -> Init_Lock/1(RunCmd)
  Unit Delay3/1 -> Calibration State/4(Closedloop_Status)
  Unit Delay1/1 -> Calibration State/3(Init_LockStatus)
  Constant3/1 -> Calibration State/2(CalibTime)
  RunCmd/1 -> Calibration State/1(RunCmd)

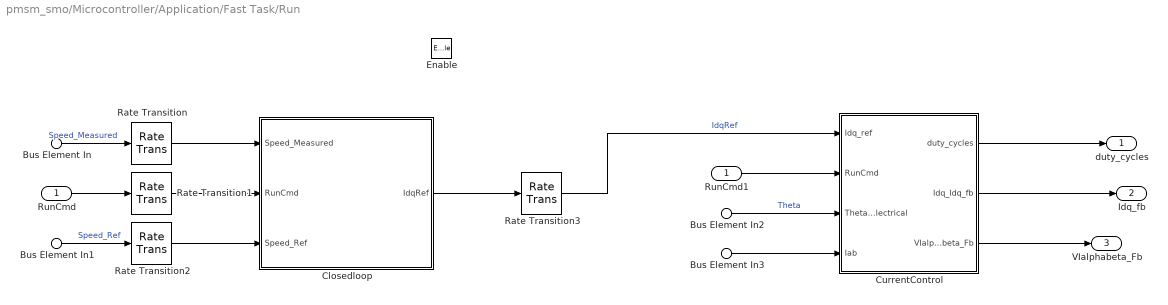
== system pmsm_smo/Microcontroller/Application/Fast Task/Run ==
  RunCmd : Inport
  Bus Element In : Inport  Port=2  PortName=HWInputs  Element=Speed_SMO
  Bus Element In1 : Inport  Port=2  PortName=HWInputs  Element=SpeedRef
  Bus Element In2 : Inport  Port=2  PortName=HWInputs  Element=Theta_SMO
  Bus Element In3 : Inport  Port=2  PortName=HWInputs  Element=Iab
  Enable : EnablePort
  Closedloop : Subsystem
  CurrentControl : Subsystem
  Rate Transition{,1..3} (4 alike) : RateTransition
  RunCmd1 : InportShadow
  duty_cycles : Outport  VectorParamsAs1DForOutWhenUnconnected=off
  Idq_fb : Outport  Port=2  VectorParamsAs1DForOutWhenUnconnected=off
  VIalphabeta_Fb : Outport  Port=3
  wires:
  Bus Element In2/1 -> CurrentControl/3(Theta_electrical)  "Theta"
  Rate Transition2/1 -> Closedloop/3(Speed_Ref)
  Rate Transition1/1 -> Closedloop/2(RunCmd)
  RunCmd1/1 -> CurrentControl/2(RunCmd)
  CurrentControl/2(Idq_Idq_fb) -> Idq_fb/1
  CurrentControl/1(duty_cycles) -> duty_cycles/1
  Closedloop/1(IdqRef) -> Rate Transition3/1
  RunCmd/1 -> Rate Transition1/1
  Rate Transition/1 -> Closedloop/1(Speed_Measured)
  Rate Transition3/1 -> CurrentControl/1(Idq_ref)  "IdqRef"
  Bus Element In3/1 -> CurrentControl/4(Iab)
  Bus Element In/1 -> Rate Transition/1  "Speed_Measured"
  Bus Element In1/1 -> Rate Transition2/1  "Speed_Ref"
  CurrentControl/3(VIalphabeta_Fb) -> VIalphabeta_Fb/1

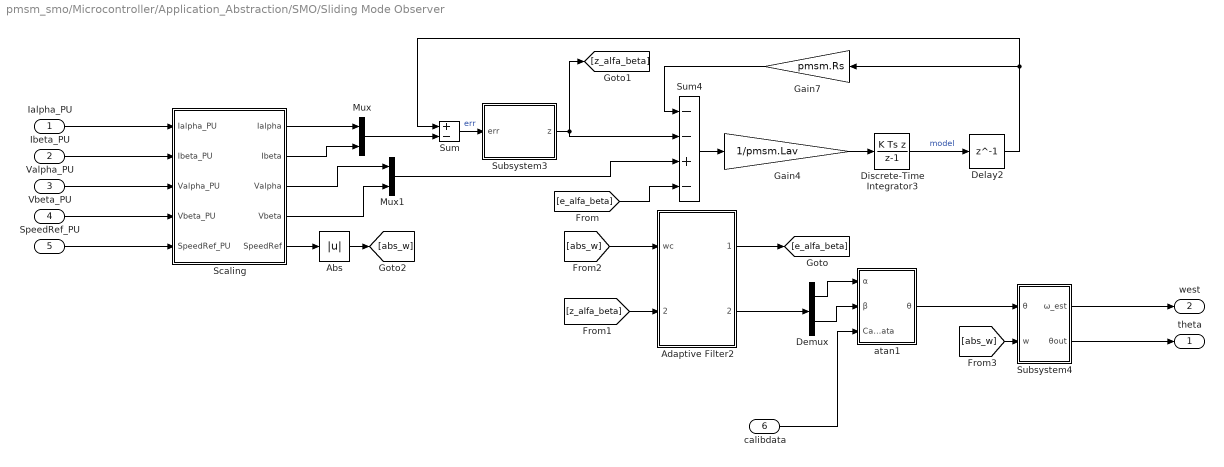
== system pmsm_smo/Microcontroller/Application_Abstraction/SMO/Sliding Mode Observer ==
  Ialpha_PU : Inport
  Ibeta_PU : Inport  Port=2
  Valpha_PU : Inport  Port=3
  Vbeta_PU : Inport  Port=4
  SpeedRef_PU : Inport  Port=5
  calibdata : Inport  Port=6
  Abs : Abs  SaturateOnIntegerOverflow=off
  Adaptive Filter2 : Subsystem
  Delay2 : Delay  DelayLength=1
  Demux : Demux  Outputs=2
  Discrete-Time Integrator3 : DiscreteIntegrator  IntegratorMethod=Integration: Backward Euler  SampleTime=-1  OutDataTypeStr=single  ICPrevOutput=DiscIntNeverNeededParam  ICPrevScaledInput=DiscIntNeverNeededParam
  Gain4 : Gain  Gain=1/pmsm.Lav  OutDataTypeStr=single
  Gain7 : Gain  Gain=pmsm.Rs  OutDataTypeStr=Inherit: Same as input
  Mux : Mux  Inputs=2
  Mux1 : Mux  Inputs=2
  Scaling : Subsystem
  Subsystem3 : Subsystem
  Subsystem4 : Subsystem
  Sum : Sum  Inputs=+-  OutDataTypeStr=single  AccumDataTypeStr=single
  Sum4 : Sum  Inputs=--+-  OutDataTypeStr=single  AccumDataTypeStr=single
  atan1 : Subsystem
  theta : Outport
  west : Outport  Port=2
  wires:
  Ialpha_PU/1 -> Scaling/1(Ialpha_PU)
  Vbeta_PU/1 -> Scaling/4(Vbeta_PU)
  Valpha_PU/1 -> Scaling/3(Valpha_PU)
  Ibeta_PU/1 -> Scaling/2(Ibeta_PU)
  SpeedRef_PU/1 -> Scaling/5(SpeedRef_PU)
  Gain7/1 -> Sum4/1
  Discrete-Time Integrator3/1 -> Delay2/1  "model"
  Sum4/1 -> Gain4/1
  Mux1/1 -> Sum4/3
  Gain4/1 -> Discrete-Time Integrator3/1
  Subsystem3/1(z) -> [z_alfa_beta], Sum4/2
  atan1/1(θ) -> Subsystem4/1(θ)
  Subsystem4/1(ω_est) -> west/1
  Sum/1 -> Subsystem3/1(err)  "err"
  Scaling/5(SpeedRef) -> Abs/1
  Scaling/1(Ialpha) -> Mux/1
  Scaling/2(Ibeta) -> Mux/2
  Scaling/3(Valpha) -> Mux1/1
  Scaling/4(Vbeta) -> Mux1/2
  [e_alfa_beta] -> Sum4/4
  Mux/1 -> Sum/2
  Delay2/1 -> Sum/1, Gain7/1
  Adaptive Filter2/1(ealfa_bita) -> [e_alfa_beta]
  Adaptive Filter2/2(ealfa_bita_fil) -> Demux/1
  [z_alfa_beta] -> Adaptive Filter2/2(zalfa_bita)
  Abs/1 -> [abs_w]
  [abs_w] -> Adaptive Filter2/1(wc)
  Demux/1 -> atan1/1(α)
  Demux/2 -> atan1/2(β)
  [abs_w] -> Subsystem4/2(w)
  Subsystem4/2(θout) -> theta/1
  calibdata/1 -> atan1/3(Calibdata)

== system pmsm_smo/Microcontroller/Command_Signals/Command Signals/Codegen ==
  Command_Data : Inport
  Data Type Conversion1 : DataTypeConversion  OutDataTypeStr=single  RndMeth=Simplest  SaturateOnIntegerOverflow=off
  Data Type Conversion4 : DataTypeConversion  OutDataTypeStr=single  RndMeth=Simplest  SaturateOnIntegerOverflow=off
  Demux : Demux  Outputs=2
  Gain1 : Gain  Gain=(2*pi/60)*pmsm.N_rated*pmsm.p
  Rate Limiter1 : RateLimiter  RisingSlewLimit=0.5  FallingSlewLimit=-0.2  SampleTimeMode=inherited
  Saturation : Saturate  UpperLimit=(2*pi/60)*pmsm.N_rated*1.5*pmsm.p  LowerLimit=(2*pi/60)*CalibSpeed*pmsm.p
  Triggered Subsystem : Subsystem  TreatAsAtomicUnit=on
  RunCmd : Outport
  SpeedRef : Outport  Port=2
  wires:
  Demux/1 -> Triggered Subsystem/Trigger
  Triggered Subsystem/1(RunCmd) -> Data Type Conversion1/1
  Gain1/1 -> Saturation/1
  Demux/2 -> Rate Limiter1/1
  Saturation/1 -> Data Type Conversion4/1
  Data Type Conversion4/1 -> SpeedRef/1
  Data Type Conversion1/1 -> RunCmd/1
  Rate Limiter1/1 -> Gain1/1
  Command_Data/1 -> Demux/1

== system pmsm_smo/Microcontroller/Command_Signals/Command Signals/Sim ==
  Command_Data : Inport
  Data Type Conversion2 : DataTypeConversion  OutDataTypeStr=single  RndMeth=Simplest  SaturateOnIntegerOverflow=off
  Data Type Conversion4 : DataTypeConversion  OutDataTypeStr=single  RndMeth=Simplest  SaturateOnIntegerOverflow=off
  Gain1 : Gain  Gain=(2*pi/60)*pmsm.N_rated*pmsm.p
  Rate Limiter3 : RateLimiter  RisingSlewLimit=0.5*(pmsm.N_rated*pmsm.p)*(2*pi/60)  FallingSlewLimit=-0.3*(pmsm.N_rated*pmsm.p)*(2*pi/60)  SampleTimeMode=inherited
  Saturation : Saturate  UpperLimit=(pmsm.N_rated*pmsm.p)*(2*pi/60)*1.5  LowerLimit=(CalibSpeed*pmsm.p)*(2*pi/60)
  Step : Step  Time=8  Before=0.1035  OutDataTypeStr=single  SampleTime=Ts
  Step1 : Step  OutDataTypeStr=single  SampleTime=Ts
  Step2 : Step  Time=8  OutDataTypeStr=single  SampleTime=Ts
  Step3 : Step  Time=9  OutDataTypeStr=single  SampleTime=Ts
  Subtract : Sum  Inputs=+-+
  Terminator : Terminator
  RunCmd : Outport
  SpeedRef : Outport  Port=2
  wires:
  Gain1/1 -> Rate Limiter3/1
  Step/1 -> Gain1/1
  Saturation/1 -> Data Type Conversion4/1
  Data Type Conversion4/1 -> SpeedRef/1
  Data Type Conversion2/1 -> RunCmd/1
  Command_Data/1 -> Terminator/1
  Rate Limiter3/1 -> Saturation/1
  Step2/1 -> Subtract/2
  Step3/1 -> Subtract/3
  Step1/1 -> Data Type Conversion2/1

== system pmsm_smo/Microcontroller/Data Monitoring/SerialInDrivers/Triggered Subsystem ==
  In1 : Inport
  Trigger : TriggerPort  VariantControl=(inherit)
  SCI_Data : Outport
  wires:
  In1/1 -> SCI_Data/1

== system pmsm_smo/Microcontroller/Data Monitoring/SerialOutDrivers/codegen ==
  SerialData : Inport
  SCI_Tx : Subsystem
  wires:
  SerialData/1 -> SCI_Tx/1(Data_Log)

== system pmsm_smo/Microcontroller/Data Monitoring/SerialOutDrivers/sim ==
  SerialData : Inport
  Terminator : Terminator
  wires:
  SerialData/1 -> Terminator/1

== system pmsm_smo/Microcontroller/Application/Fast Task/Prepare/Init_Lock ==
  RunCmd : Inport
  Enable : EnablePort
  Compare To Constant1 : simulink/Logic and Bit Operations/Compare To Constant  relop===  const=1  OutDataTypeStr=boolean
  Compare To Constant2 : simulink/Logic and Bit Operations/Compare To Constant  relop===  const=0  OutDataTypeStr=boolean
  Compare To Constant3 : simulink/Logic and Bit Operations/Compare To Constant  relop===  const=2  OutDataTypeStr=boolean
  Init : Subsystem
  Lock : Subsystem
  Multiport Switch1 : MultiPortSwitch  DataPortOrder=Zero-based contiguous  DiagnosticForDefault=None  zeroidx=on  OutDataTypeStr=single  SaturateOnIntegerOverflow=off  InputSameDT=off
  Rotor Locking : Stateflow chart  TreatAsAtomicUnit=on
  Theta_Calib : Subsystem
  duty_cycles : Outport  VectorParamsAs1DForOutWhenUnconnected=off
  Init_LockStatus : Outport  Port=2
  wires:
  Compare To Constant1/1 -> Lock/Enable
  Compare To Constant2/1 -> Init/Enable
  Compare To Constant3/1 -> Theta_Calib/Enable
  Theta_Calib/1(Vabc) -> Multiport Switch1/4
  Multiport Switch1/1 -> duty_cycles/1  "Vabc"
  [Lock] -> Multiport Switch1/1
  Init/1(Vabc) -> Multiport Switch1/2
  Lock/1(duty_cycles) -> Multiport Switch1/3
  Rotor Locking/1(Lock) -> Compare To Constant1/1, Compare To Constant3/1, Compare To Constant2/1, [Lock]
  Rotor Locking/2(Init_LockStatus) -> Init_LockStatus/1
  RunCmd/1 -> Rotor Locking/1(RunCmd)

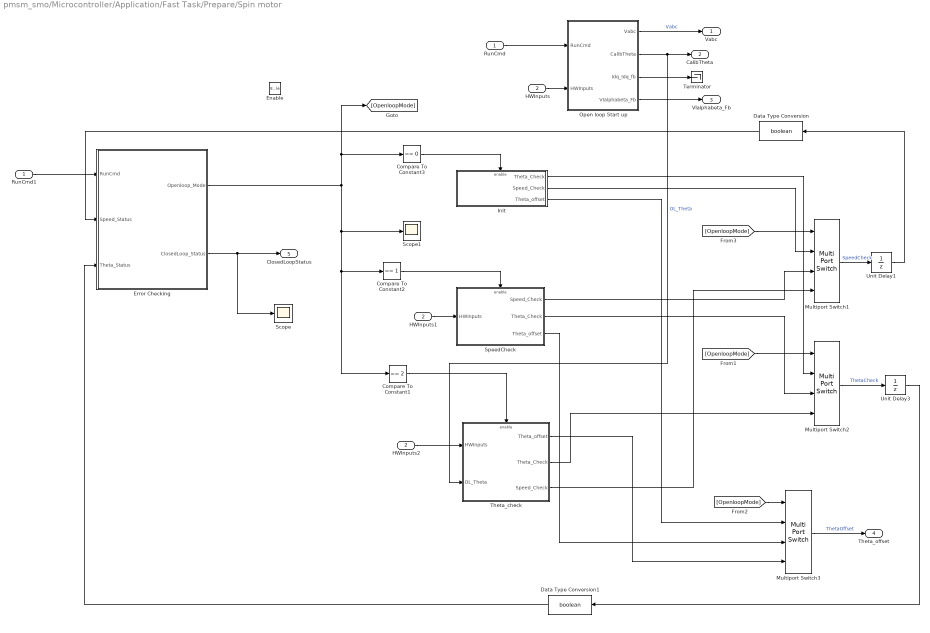
== system pmsm_smo/Microcontroller/Application/Fast Task/Prepare/Spin motor ==
  RunCmd : Inport
  HWInputs : Inport  Port=2
  Enable : EnablePort
  Compare To Constant1 : simulink/Logic and Bit Operations/Compare To Constant  relop===  const=2  OutDataTypeStr=boolean
  Compare To Constant2 : simulink/Logic and Bit Operations/Compare To Constant  relop===  const=1  OutDataTypeStr=boolean
  Compare To Constant3 : simulink/Logic and Bit Operations/Compare To Constant  relop===  const=0  OutDataTypeStr=boolean
  Data Type Conversion : DataTypeConversion  OutDataTypeStr=boolean  ConvertRealWorld=Stored Integer (SI)  SaturateOnIntegerOverflow=off  RndMeth=Floor
  Data Type Conversion1 : DataTypeConversion  OutDataTypeStr=boolean  ConvertRealWorld=Stored Integer (SI)  SaturateOnIntegerOverflow=off  RndMeth=Floor
  Error Checking : Stateflow chart  TreatAsAtomicUnit=on
  HWInputs1 : InportShadow  Port=2
  HWInputs2 : InportShadow  Port=2
  Init : Subsystem
  Multiport Switch1 : MultiPortSwitch  DataPortOrder=Zero-based contiguous  DiagnosticForDefault=None  zeroidx=on  OutDataTypeStr=single  SaturateOnIntegerOverflow=off  InputSameDT=off
  Multiport Switch2 : MultiPortSwitch  DataPortOrder=Zero-based contiguous  DiagnosticForDefault=None  zeroidx=on  OutDataTypeStr=single  SaturateOnIntegerOverflow=off  InputSameDT=off
  Multiport Switch3 : MultiPortSwitch  DataPortOrder=Zero-based contiguous  DiagnosticForDefault=None  zeroidx=on  OutDataTypeStr=single  SaturateOnIntegerOverflow=off  InputSameDT=off
  Open loop Start up : Subsystem
  RunCmd1 : InportShadow
  Scope : Scope
  Scope1 : Scope
  SpeedCheck : Subsystem
  Terminator : Terminator
  Theta_check : Subsystem
  Unit Delay1 : UnitDelay  SampleTime=Ts  HasFrameUpgradeWarning=on
  Unit Delay3 : UnitDelay  SampleTime=Ts  HasFrameUpgradeWarning=on
  Vabc : Outport  VectorParamsAs1DForOutWhenUnconnected=off
  CalibTheta : Outport  Port=2
  VIalphabeta_Fb : Outport  Port=3
  Theta_offset : Outport  Port=4
  ClosedLoopStatus : Outport  Port=5
  wires:
  Open loop Start up/1(Vabc) -> Vabc/1  "Vabc"
  Open loop Start up/2(CalibTheta) -> CalibTheta/1, Theta_check/2(OL_Theta)  "OL_Theta"
  Open loop Start up/3(Idq_Idq_fb) -> Terminator/1
  RunCmd/1 -> Open loop Start up/1(RunCmd)
  Open loop Start up/4(VIalphabeta_Fb) -> VIalphabeta_Fb/1
  Error Checking/1(Openloop_Mode) -> Scope1/1, Compare To Constant1/1, Compare To Constant2/1, [OpenloopMode], Compare To Constant3/1
  Compare To Constant2/1 -> SpeedCheck/Enable
  Compare To Constant1/1 -> Theta_check/Enable
  RunCmd1/1 -> Error Checking/1(RunCmd)
  HWInputs/1 -> Open loop Start up/2(HWInputs)
  HWInputs2/1 -> Theta_check/1(HWInputs)
  HWInputs1/1 -> SpeedCheck/1(HWInputs)
  Error Checking/2(ClosedLoop_Status) -> Scope/1, ClosedLoopStatus/1
  Compare To Constant3/1 -> Init/Enable
  SpeedCheck/1(Speed_Check) -> Multiport Switch1/3
  Theta_check/3(Speed_Check) -> Multiport Switch1/4
  Multiport Switch1/1 -> Unit Delay1/1  "SpeedCheck"
  Init/2(Speed_Check) -> Multiport Switch1/2
  [OpenloopMode] -> Multiport Switch1/1
  Unit Delay1/1 -> Data Type Conversion/1
  SpeedCheck/2(Theta_Check) -> Multiport Switch2/3
  Theta_check/2(Theta_Check) -> Multiport Switch2/4
  [OpenloopMode] -> Multiport Switch2/1
  Init/1(Theta_Check) -> Multiport Switch2/2
  Multiport Switch2/1 -> Unit Delay3/1  "ThetaCheck"
  Unit Delay3/1 -> Data Type Conversion1/1
  Theta_check/1(Theta_offset) -> Multiport Switch3/4
  [OpenloopMode] -> Multiport Switch3/1
  SpeedCheck/3(Theta_offset) -> Multiport Switch3/3
  Init/3(Theta_offset) -> Multiport Switch3/2
  Multiport Switch3/1 -> Theta_offset/1  "ThetaOffset"
  Data Type Conversion/1 -> Error Checking/2(Speed_Status)
  Data Type Conversion1/1 -> Error Checking/3(Theta_Status)

== system pmsm_smo/Microcontroller/Application/Fast Task/Run/Closedloop ==
  Speed_Measured : Inport
  RunCmd : Inport  Port=2
  Speed_Ref : Inport  Port=3
  Speed Control : Subsystem  TreatAsAtomicUnit=on  SystemSampleTime=Ts_speed
  IdqRef : Outport
  wires:
  RunCmd/1 -> Speed Control/2(RunCmd)
  Speed_Ref/1 -> Speed Control/3(Speed_Ref)
  Speed_Measured/1 -> Speed Control/1(Speed_Meas)
  Speed Control/1(IdqRef) -> IdqRef/1

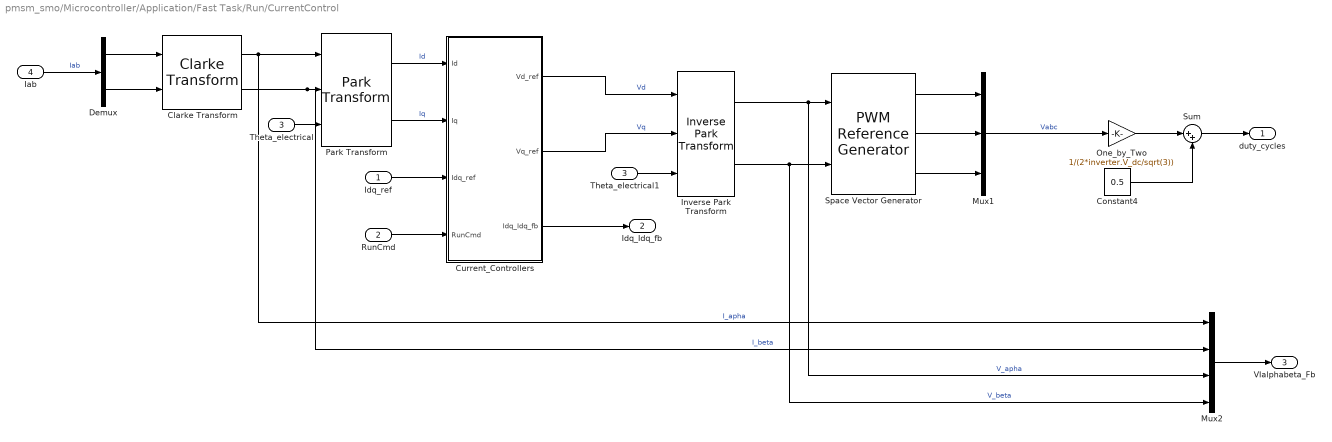
== system pmsm_smo/Microcontroller/Application/Fast Task/Run/CurrentControl ==
  Idq_ref : Inport
  RunCmd : Inport  Port=2
  Theta_electrical : Inport  Port=3
  Iab : Inport  Port=4
  Clarke Transform : mcbcontrolslib/Clarke Transform  VariantControl=Variant2  PhaseInput=Two inputs  EnPowerInv=off
  Constant4 : Constant  Value=0.5  OutDataTypeStr=dataType  SampleTime=-1
  Current_Controllers : Subsystem
  Demux : Demux  Outputs=2
  Inverse Park Transform : mcbcontrolslib/Inverse Park Transform  PhaseInput=Two inputs  AxisAlignment=D-axis  ThetaInput=Electrical position  AngleInput=Radians  N_points=1024
  Mux1 : Mux  Inputs=3
  Mux2 : Mux
  One_by_Two : Gain  Gain=1/(2*inverter.V_dc/sqrt(3))  RndMeth=Simplest  OutDataTypeStr=Inherit: Same as input
  Park Transform : mcbcontrolslib/Park Transform  PhaseInput=Two inputs  AxisAlignment=D-axis  ThetaInput=Electrical position  AngleInput=Radians  N_points=1024
  Space Vector Generator : mcbcontrolslib/PWM Reference Generator  inSignal=Valphabeta  modType=SVM: space vector modulation
  Sum : Sum  Inputs=|++
  Theta_electrical1 : InportShadow  Port=3
  duty_cycles : Outport  VectorParamsAs1DForOutWhenUnconnected=off
  Idq_Idq_fb : Outport  Port=2  VectorParamsAs1DForOutWhenUnconnected=off
  VIalphabeta_Fb : Outport  Port=3
  wires:
  Park Transform/1 -> Current_Controllers/1(Id)  "Id"
  Space Vector Generator/3 -> Mux1/3
  Space Vector Generator/1 -> Mux1/1
  Space Vector Generator/2 -> Mux1/2
  Current_Controllers/1(Vd_ref) -> Inverse Park Transform/1  "Vd"
  One_by_Two/1 -> Sum/1
  Park Transform/2 -> Current_Controllers/2(Iq)  "Iq"
  Current_Controllers/3(Idq_Idq_fb) -> Idq_Idq_fb/1
  Constant4/1 -> Sum/2
  Idq_ref/1 -> Current_Controllers/3(Idq_ref)
  Mux1/1 -> One_by_Two/1  "Vabc"
  Sum/1 -> duty_cycles/1
  Current_Controllers/2(Vq_ref) -> Inverse Park Transform/2  "Vq"
  RunCmd/1 -> Current_Controllers/4(RunCmd)
  Iab/1 -> Demux/1  "Iab"
  Theta_electrical/1 -> Park Transform/3
  Theta_electrical1/1 -> Inverse Park Transform/3
  Demux/1 -> Clarke Transform/1
  Demux/2 -> Clarke Transform/2
  Clarke Transform/1 -> Park Transform/1, Mux2/1  "I_apha"
  Clarke Transform/2 -> Park Transform/2, Mux2/2  "I_beta"
  Mux2/1 -> VIalphabeta_Fb/1
  Inverse Park Transform/1 -> Mux2/3, Space Vector Generator/1  "V_apha"
  Inverse Park Transform/2 -> Mux2/4, Space Vector Generator/2  "V_beta"

== system pmsm_smo/Microcontroller/Application_Abstraction/SMO/Sliding Mode Observer/Adaptive Filter2 ==
  wc : Inport
  zalfa_bita : Inport  Port=2
  Delay : Delay  DelayLength=1
  Delay3 : Delay  DelayLength=1
  Discrete-Time Integrator : DiscreteIntegrator  IntegratorMethod=Integration: Backward Euler  SampleTime=-1  OutDataTypeStr=single  ICPrevOutput=DiscIntNeverNeededParam  ICPrevScaledInput=DiscIntNeverNeededParam
  Discrete-Time Integrator2 : DiscreteIntegrator  IntegratorMethod=Integration: Backward Euler  SampleTime=-1  OutDataTypeStr=single  ICPrevOutput=DiscIntNeverNeededParam  ICPrevScaledInput=DiscIntNeverNeededParam
  Product : Product  OutDataTypeStr=single
  Product2 : Product  OutDataTypeStr=single
  Sum2 : Sum  Inputs=|+-  OutDataTypeStr=Inherit: Same as first input
  Sum3 : Sum  Inputs=|+-  OutDataTypeStr=single  AccumDataTypeStr=single
  ealfa_bita : Outport  VectorParamsAs1DForOutWhenUnconnected=off
  ealfa_bita_fil : Outport  Port=2  VectorParamsAs1DForOutWhenUnconnected=off
  wires:
  Sum2/1 -> Product/2
  Product/1 -> Discrete-Time Integrator/1
  Product2/1 -> Discrete-Time Integrator2/1
  Sum3/1 -> Product2/2
  zalfa_bita/1 -> Sum2/1
  Delay/1 -> Sum2/2
  Delay3/1 -> Sum3/2
  wc/1 -> Product/1, Product2/1
  Discrete-Time Integrator2/1 -> ealfa_bita_fil/1, Delay3/1
  Discrete-Time Integrator/1 -> Delay/1, ealfa_bita/1, Sum3/1

== system pmsm_smo/Microcontroller/Application_Abstraction/SMO/Sliding Mode Observer/Scaling ==
  Ialpha_PU : Inport
  Ibeta_PU : Inport  Port=2
  Valpha_PU : Inport  Port=3
  Vbeta_PU : Inport  Port=4
  SpeedRef_PU : Inport  Port=5
  Ialpha : Outport
  Ibeta : Outport  Port=2
  Valpha : Outport  Port=3
  Vbeta : Outport  Port=4
  SpeedRef : Outport  Port=5
  wires:
  Ibeta_PU/1 -> Ibeta/1
  Valpha_PU/1 -> Valpha/1
  Vbeta_PU/1 -> Vbeta/1
  Ialpha_PU/1 -> Ialpha/1
  SpeedRef_PU/1 -> SpeedRef/1

== system pmsm_smo/Microcontroller/Application_Abstraction/SMO/Sliding Mode Observer/Subsystem3 ==
  err : Inport
  Abs1 : Abs  SaturateOnIntegerOverflow=off
  Compare To Constant1 : simulink/Logic and Bit Operations/Compare To Constant  relop=>=  const=1.14  OutDataTypeStr=boolean
  Gain4 : Gain  Gain=7.5512  OutDataTypeStr=single
  Gain7 : Gain  Gain=8.61  OutDataTypeStr=single
  Sign1 : Signum
  Switch1 : Switch  Criteria=u2 > Threshold  SaturateOnIntegerOverflow=off  InputSameDT=off  OutDataTypeStr=Inherit: Same as first input
  z : Outport
  wires:
  Switch1/1 -> z/1
  Gain4/1 -> Switch1/3  "z"
  Abs1/1 -> Compare To Constant1/1
  Gain7/1 -> Switch1/1
  Compare To Constant1/1 -> Switch1/2
  err/1 -> Gain4/1, Abs1/1, Sign1/1
  Sign1/1 -> Gain7/1  "z"

== system pmsm_smo/Microcontroller/Application_Abstraction/SMO/Sliding Mode Observer/Subsystem4 ==
  θ : Inport
  w : Inport  Port=2
  Delay1 : Delay  DelayLength=1
  Discrete-Time Integrator4 : DiscreteIntegrator  IntegratorMethod=Integration: Backward Euler  SampleTime=-1  OutDataTypeStr=single  ICPrevOutput=DiscIntNeverNeededParam  ICPrevScaledInput=DiscIntNeverNeededParam
  Gain2 : Gain  Gain=0.3  OutDataTypeStr=single
  Gain3 : Gain  Gain=1/Ts  OutDataTypeStr=single
  Product1 : Product  OutDataTypeStr=single
  Sum2 : Sum  Inputs=|+-  OutDataTypeStr=single  AccumDataTypeStr=single
  Sum4 : Sum  Inputs=|+-  OutDataTypeStr=Inherit: Same as first input
  Unit Delay3 : UnitDelay  SampleTime=Ts  HasFrameUpgradeWarning=on
  Wrap_to_pi1 : Subsystem  VariantControl=VSS_STD
  Wrap_to_pi2 : Subsystem  VariantControl=VSS_STD
  ω_est : Outport  VectorParamsAs1DForOutWhenUnconnected=off
  θout : Outport  Port=2  VectorParamsAs1DForOutWhenUnconnected=off
  wires:
  Unit Delay3/1 -> Sum2/2
  θ/1 -> Wrap_to_pi1/1(θ), Sum2/1, Unit Delay3/1
  Sum4/1 -> Product1/2
  Product1/1 -> Discrete-Time Integrator4/1
  Delay1/1 -> Sum4/2
  Sum2/1 -> Wrap_to_pi2/1(θ)
  Discrete-Time Integrator4/1 -> ω_est/1, Delay1/1
  w/1 -> Gain2/1
  Gain2/1 -> Product1/1
  Gain3/1 -> Sum4/1
  Wrap_to_pi2/1(θ (-π,π)) -> Gain3/1
  Wrap_to_pi1/1(θ (-π,π)) -> θout/1
